simulink subsystem "HI_VectorBox"  (R2019b)
settings: Solver=VariableStepAuto  StartTime=0.0  StopTime=10.0  RelTol=1e-3
libraries: canmsglib x1, c280xlib x1
settings Model: Creator=Nick  LastModifiedBy=Nick

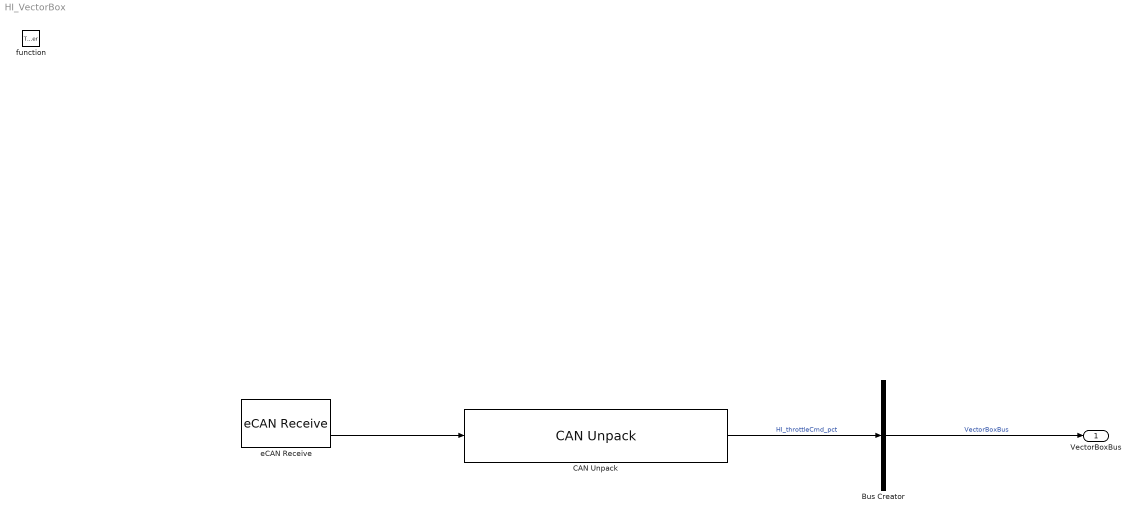
== system HI_VectorBox ==
  function : TriggerPort  TriggerType=function-call  VariantControl=Variant
  Bus Creator : BusCreator  Inputs=1
  CAN Unpack : canmsglib/CAN Unpack  CANdbFile=C:\Git\ETC-Development\DBCs\F28377S_etc_benchTest.dbc  MsgList=ETC_adcRaw1  MsgName=VBOX_cmd1  MsgIDType=Standard (11-bit identifier)  MsgIdentifier=500  MsgLength=2  SignalInfo={ 'VBOX_throttleCmd', '0', '16', 'LE', 'signed', 'Standard', '0', '0.01', '0', '-327.68', '327.67' }  IDPort=off  TimestampPort=off  ErrorPort=off  RemotePort=off  LengthPort=off  StatusPort=off  ApplyMinMax=off
      settings: SourceProductName=Vehicle Network Toolbox  SourceProductBaseCode=VN  DataFormat=CANdb specified signals
  eCAN Receive : c280xlib/eCAN Receive  chipFamily=C280x  useModule=eCAN_A  mailboxNo=11  messageID=500  messageType=Standard (11-bit identifier)  sampleTime=-1  dataType=CAN_MESSAGE_TYPE  initValue=0  outputMessageLength=off  outputMessageTimeStamp=off  postInterrupt=off  interruptLine=0
      settings: SourceProductName=Embedded Coder Support Package for Texas Instruments C2000 Processors  SourceProductBaseCode=TIC2000
  VectorBoxBus : Outport
  wires:
  CAN Unpack/1 -> Bus Creator/1  "HI_throttleCmd_pct"
  eCAN Receive/2 -> CAN Unpack/1
  Bus Creator/1 -> VectorBoxBus/1  "VectorBoxBus"
